simulink model "ornithopter_model"  (R2019a)
settings: Solver=VariableStepAuto  StartTime=0.0  StopTime=10.0  RelTol=1e-3
settings Model: Creator=rinku  LastModifiedBy=rinku

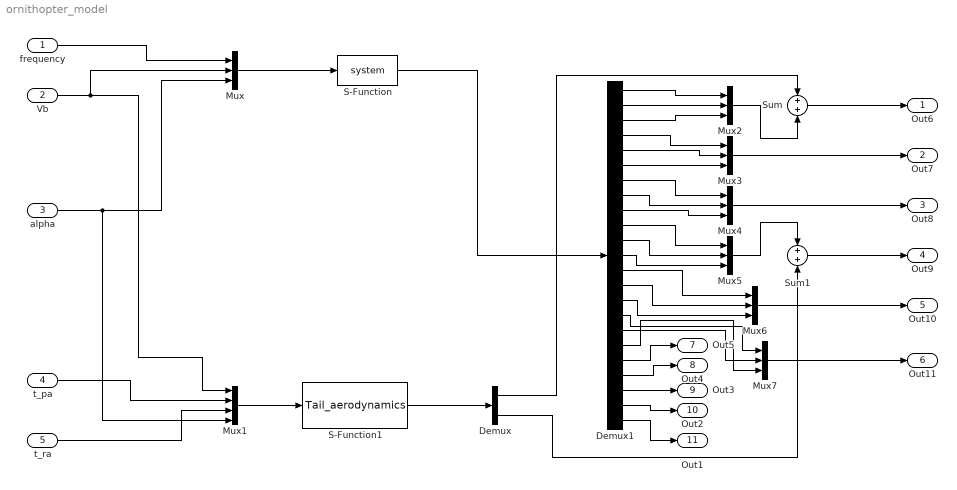
== system ornithopter_model ==
  frequency : Inport
  Vb : Inport  Port=2
  alpha : Inport  Port=3
  t_pa : Inport  Port=4
  t_ra : Inport  Port=5
  Demux : Demux  Outputs=2
  Demux1 : Demux  Outputs=23
  Mux{,2..7} (7 alike) : Mux  Inputs=3
  Mux1 : Mux
  S-Function : S-Function  SFunctionDeploymentMode=off  EnableBusSupport=off
  S-Function1 : S-Function  FunctionName=Tail_aerodynamics  SFunctionDeploymentMode=off  EnableBusSupport=off
  Sum : Sum  Inputs=2
  Sum1 : Sum  Inputs=2
  Out6 : Outport
  Out7 : Outport  Port=2
  Out8 : Outport  Port=3
  Out9 : Outport  Port=4
  Out10 : Outport  Port=5
  Out11 : Outport  Port=6
  Out5 : Outport  Port=7
  Out4 : Outport  Port=8
  Out3 : Outport  Port=9
  Out2 : Outport  Port=10
  Out1 : Outport  Port=11
  wires:
  frequency/1 -> Mux/1
  Vb/1 -> Mux1/1, Mux/2
  t_pa/1 -> Mux1/2
  t_ra/1 -> Mux1/3
  alpha/1 -> Mux1/4, Mux/3
  Mux/1 -> S-Function/1
  Mux1/1 -> S-Function1/1
  S-Function1/1 -> Demux/1
  Demux1/23 -> Out1/1
  Demux1/22 -> Out2/1
  Demux1/21 -> Out3/1
  Demux1/20 -> Out4/1
  Demux1/19 -> Out5/1
  Demux1/1 -> Mux2/1
  Demux1/2 -> Mux2/2
  Demux1/3 -> Mux2/3
  Demux1/4 -> Mux3/1
  Demux1/5 -> Mux3/2
  Demux1/6 -> Mux3/3
  Demux1/7 -> Mux4/1
  Demux1/8 -> Mux4/2
  Demux1/9 -> Mux4/3
  Demux1/10 -> Mux5/1
  Demux1/11 -> Mux5/2
  Demux1/12 -> Mux5/3
  Demux1/13 -> Mux6/1
  Demux1/14 -> Mux6/2
  Demux1/15 -> Mux6/3
  Demux1/16 -> Mux7/1
  Demux1/17 -> Mux7/2
  Demux1/18 -> Mux7/3
  Mux2/1 -> Sum/2
  Demux/1 -> Sum/1
  Demux/2 -> Sum1/2
  Mux7/1 -> Out11/1
  Mux6/1 -> Out10/1
  Mux5/1 -> Sum1/1
  Sum1/1 -> Out9/1
  Mux4/1 -> Out8/1
  Mux3/1 -> Out7/1
  Sum/1 -> Out6/1
  S-Function/1 -> Demux1/1
